simulink model "GitAffineFormationDelayInput"  (R2020b)
settings: Solver=ode4  StartTime=0.0  StopTime=50  FixedStep=0.01  RelTol=1e-3
(part 1 of 2)
settings Model: Creator=Fitz  LastModifiedBy=Fitz
settings DebuggingCC: UnderSpecifiedDimensionMsg=warning

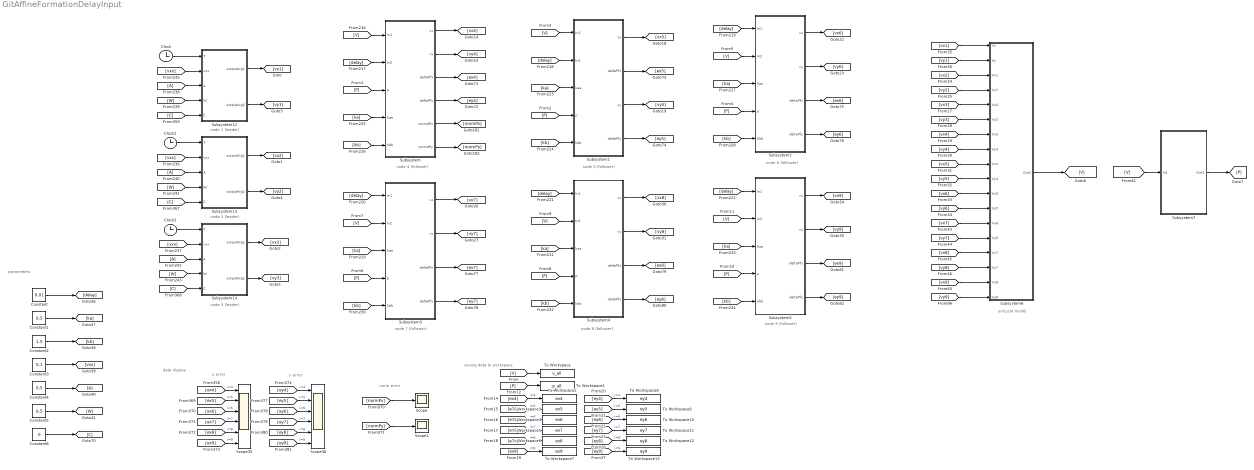
== system GitAffineFormationDelayInput ==
  note: unicycle model
  note: norm error
  note: y error
  note: x error
  note: node 1 (leader)
  note: data display
  note: parameters
  note: node 2 (leader)
  note: node 3 (leader)
  note: node 4 (follower)
  note: node 7 (follower)
  note: node 5 (follower)
  note: node 8 (follower)
  note: node 9 (follower)
  note: node 6 (follower)
  note: saving data to
      | workspace
  Clock : Clock
      settings: Decimation=100
  Clock1 : Clock
      settings: Decimation=100
  Clock2 : Clock
      settings: Decimation=100
  Constant : Constant  Value=0.01
  Constant1 : Constant  Value=0.5
  Constant2 : Constant  Value=1.5
  Constant3 : Constant  Value=0.1
  Constant4 : Constant  Value=0.5
  Constant5 : Constant  Value=0.5
  Constant6 : Constant  Value=0
  Scope : Scope
  Scope1 : Scope
  Scope35 : Scope  NumInputPorts=6
  Scope36 : Scope  NumInputPorts=6
  Subsystem : Subsystem
  Subsystem1 : Subsystem
  Subsystem12 : Subsystem
  Subsystem13 : Subsystem
  Subsystem14 : Subsystem
  Subsystem2 : Subsystem
  Subsystem3 : Subsystem
  Subsystem4 : Subsystem
  Subsystem5 : Subsystem
  Subsystem6 : Subsystem
  Subsystem7 : Subsystem
  To Workspace : ToWorkspace  VariableName=v_all  SaveFormat=Timeseries  SampleTime=-1
  To Workspace1 : ToWorkspace  VariableName=p_all  SaveFormat=Timeseries  SampleTime=-1
  To Workspace10 : ToWorkspace  VariableName=ey6  SaveFormat=Timeseries  SampleTime=-1
  To Workspace11 : ToWorkspace  VariableName=ey7  SaveFormat=Timeseries  SampleTime=-1
  To Workspace12 : ToWorkspace  VariableName=ey8  SaveFormat=Timeseries  SampleTime=-1
  To Workspace13 : ToWorkspace  VariableName=ey9  SaveFormat=Timeseries  SampleTime=-1
  To Workspace2 : ToWorkspace  VariableName=ex4  SaveFormat=Timeseries  SampleTime=-1
  To Workspace3 : ToWorkspace  VariableName=ex5  SaveFormat=Timeseries  SampleTime=-1
  To Workspace4 : ToWorkspace  VariableName=ex6  SaveFormat=Timeseries  SampleTime=-1
  To Workspace5 : ToWorkspace  VariableName=ex7  SaveFormat=Timeseries  SampleTime=-1
  To Workspace6 : ToWorkspace  VariableName=ex8  SaveFormat=Timeseries  SampleTime=-1
  To Workspace7 : ToWorkspace  VariableName=ex9  SaveFormat=Timeseries  SampleTime=-1
  To Workspace8 : ToWorkspace  VariableName=ey4  SaveFormat=Timeseries  SampleTime=-1
  To Workspace9 : ToWorkspace  VariableName=ey5  SaveFormat=Timeseries  SampleTime=-1
  wires:
  Constant/1 -> [delay]
  Constant1/1 -> [ka]
  Constant2/1 -> [kb]
  Constant3/1 -> [vxx]
  Constant4/1 -> [A]
  Constant5/1 -> [W]
  Constant6/1 -> [C]
  [ex4] -> Scope35/1  "i=4"
  [ex5] -> Scope35/2  "i=5"
  [ex6] -> Scope35/3  "i=6"
  [ex7] -> Scope35/4  "i=7"
  [ex8] -> Scope35/5  "i=8"
  [ex9] -> Scope35/6  "i=9"
  [ey9] -> Scope36/6  "i=9"
  [ey7] -> Scope36/4  "i=7"
  [ey5] -> Scope36/2  "i=5"
  [ey6] -> Scope36/3  "i=6"
  [ey8] -> Scope36/5  "i=8"
  [ey4] -> Scope36/1  "i=4"
  [V] -> Subsystem/1(In1)
  [delay] -> Subsystem/2(In2)
  [P] -> Subsystem/3(p)
  [ka] -> Subsystem/4(kaa)
  [kb] -> Subsystem/5(kbb)
  Subsystem/1(vx) -> [vx4]
  Subsystem/2(vy) -> [vy4]
  Subsystem/3(deltaPfx) -> [ex4]
  Subsystem/4(deltaPfy) -> [ey4]
  Subsystem/5(normdPx) -> [normPx]
  Subsystem/6(normdPy) -> [normPy]
  [V] -> Subsystem1/1(In1)
  [delay] -> Subsystem1/2(In2)
  [ka] -> Subsystem1/3(kaa)
  [P] -> Subsystem1/4(p)
  [kb] -> Subsystem1/5(kbb)
  Subsystem1/1(vx) -> [vx5]
  Subsystem1/2(deltaPfx) -> [ex5]
  Subsystem1/3(vy) -> [vy5]
  Subsystem1/4(deltaPfy) -> [ey5]
  [delay] -> Subsystem2/1(In1)
  [V] -> Subsystem2/2(In2)
  [ka] -> Subsystem2/3(kaa)
  [P] -> Subsystem2/4(p)
  [kb] -> Subsystem2/5(kbb)
  Subsystem2/1(vx) -> [vx6]
  Subsystem2/2(vy) -> [vy6]
  Subsystem2/3(deltaPfx) -> [ex6]
  Subsystem2/4(deltaPfy) -> [ey6]
  [delay] -> Subsystem3/1(In1)
  [V] -> Subsystem3/2(In2)
  [ka] -> Subsystem3/3(kaa)
  [P] -> Subsystem3/4(p)
  [kb] -> Subsystem3/5(kbb)
  Subsystem3/1(vx) -> [vx7]
  Subsystem3/2(vy) -> [vy7]
  Subsystem3/3(deltaPfx) -> [ex7]
  Subsystem3/4(deltaPfy) -> [ey7]
  [delay] -> Subsystem4/1(In1)
  [V] -> Subsystem4/2(In2)
  [ka] -> Subsystem4/3(kaa)
  [P] -> Subsystem4/4(p)
  [kb] -> Subsystem4/5(kbb)
  Subsystem4/1(vx) -> [vx8]
  Subsystem4/2(vy) -> [vy8]
  Subsystem4/3(deltaPfx) -> [ex8]
  Subsystem4/4(deltaPfy) -> [ey8]
  [delay] -> Subsystem5/1(In1)
  [V] -> Subsystem5/2(In2)
  [ka] -> Subsystem5/3(kaa)
  [P] -> Subsystem5/4(p)
  [kb] -> Subsystem5/5(kbb)
  Subsystem5/1(vx) -> [vx9]
  Subsystem5/2(vy) -> [vy9]
  Subsystem5/3(deltaPfx) -> [ex9]
  Subsystem5/4(deltaPfy) -> [ey9]
  Clock/1 -> Subsystem12/1(T)
  [vxx] -> Subsystem12/2(vxx)
  [A] -> Subsystem12/3(A)
  [W] -> Subsystem12/4(W)
  [C] -> Subsystem12/5(C)
  Subsystem12/1(outputArg1) -> [vx1]
  Subsystem12/2(outputArg2) -> [vy1]
  Clock1/1 -> Subsystem13/1(T)
  [vxx] -> Subsystem13/2(vxx)
  [A] -> Subsystem13/3(A)
  [W] -> Subsystem13/4(W)
  [C] -> Subsystem13/5(C)
  Subsystem13/1(outputArg1) -> [vx2]
  Subsystem13/2(outputArg2) -> [vy2]
  Clock2/1 -> Subsystem14/1(T)
  [vxx] -> Subsystem14/2(vxx)
  [A] -> Subsystem14/3(A)
  [W] -> Subsystem14/4(W)
  [C] -> Subsystem14/5(C)
  Subsystem14/1(outputArg1) -> [vx3]
  Subsystem14/2(outputArg2) -> [vy3]
  [normPx] -> Scope/1
  [normPy] -> Scope1/1
  [V] -> To Workspace/1
  [P] -> To Workspace1/1
  [ex4] -> To Workspace2/1  "i=4"
  [ex9] -> To Workspace7/1  "i=9"
  [ex8] -> To Workspace6/1  "i=8"
  [ex6] -> To Workspace4/1  "i=6"
  [ex5] -> To Workspace3/1  "i=5"
  [ex7] -> To Workspace5/1  "i=7"
  [ey4] -> To Workspace8/1  "i=4"
  [ey9] -> To Workspace13/1  "i=9"
  [ey8] -> To Workspace12/1  "i=8"
  [ey5] -> To Workspace9/1  "i=5"
  [ey6] -> To Workspace10/1  "i=6"
  [ey7] -> To Workspace11/1  "i=7"
  [vx1] -> Subsystem6/1(Vx)
  [vy1] -> Subsystem6/2(Vy)
  [vx2] -> Subsystem6/3(Vx1)
  [vy2] -> Subsystem6/4(Vy1)
  [vx3] -> Subsystem6/5(Vx2)
  [vy3] -> Subsystem6/6(Vy2)
  [vx4] -> Subsystem6/7(Vx3)
  [vy4] -> Subsystem6/8(Vy3)
  [vx5] -> Subsystem6/9(Vx4)
  [vy5] -> Subsystem6/10(Vy4)
  [vx6] -> Subsystem6/11(Vx5)
  [vy6] -> Subsystem6/12(Vy5)
  [vx7] -> Subsystem6/13(Vx6)
  [vy7] -> Subsystem6/14(Vy6)
  [vx8] -> Subsystem6/15(Vx7)
  [vy8] -> Subsystem6/16(Vy7)
  [vx9] -> Subsystem6/17(Vx8)
  [vy9] -> Subsystem6/18(Vy8)
  Subsystem6/1(Out1) -> [V]
  [V] -> Subsystem7/1(In1)
  Subsystem7/1(Out1) -> [P]

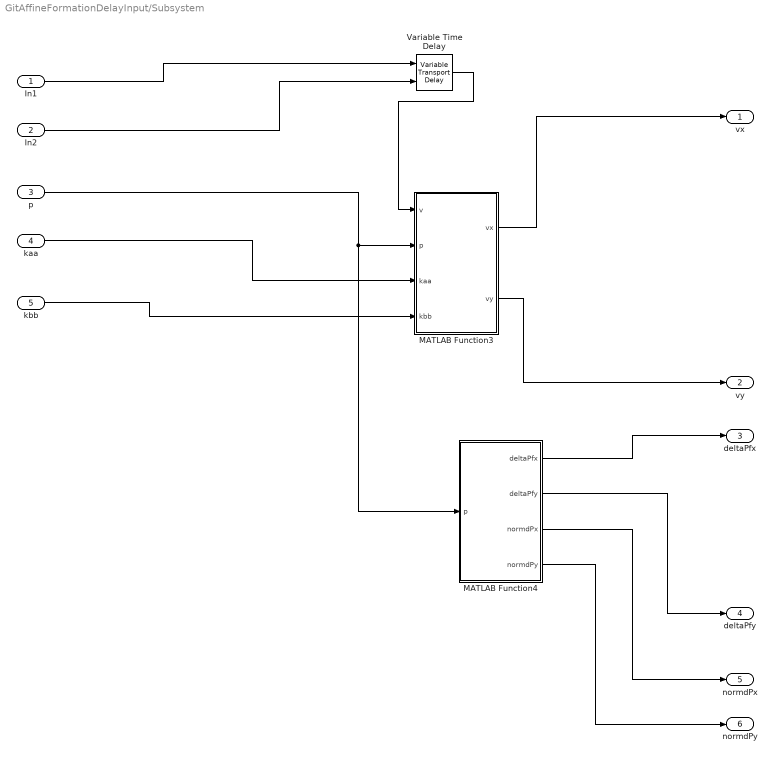
== system GitAffineFormationDelayInput/Subsystem ==
  In1 : Inport
  In2 : Inport  Port=2
  p : Inport  Port=3
  kaa : Inport  Port=4
  kbb : Inport  Port=5
  MATLAB Function3 : MATLAB Function  TreatAsAtomicUnit=on
  MATLAB Function4 : MATLAB Function  TreatAsAtomicUnit=on
  Variable Time Delay : VariableTransportDelay  MaximumDelay=10
  vx : Outport
  vy : Outport  Port=2
  deltaPfx : Outport  Port=3
  deltaPfy : Outport  Port=4
  normdPx : Outport  Port=5
  normdPy : Outport  Port=6
  wires:
  MATLAB Function4/2(deltaPfy) -> deltaPfy/1
  MATLAB Function4/1(deltaPfx) -> deltaPfx/1
  MATLAB Function3/2(vy) -> vy/1
  MATLAB Function3/1(vx) -> vx/1
  p/1 -> MATLAB Function4/1(p), MATLAB Function3/2(p)
  MATLAB Function4/3(normdPx) -> normdPx/1
  Variable Time Delay/1 -> MATLAB Function3/1(v)
  MATLAB Function4/4(normdPy) -> normdPy/1
  kbb/1 -> MATLAB Function3/4(kbb)
  In2/1 -> Variable Time Delay/2
  kaa/1 -> MATLAB Function3/3(kaa)
  In1/1 -> Variable Time Delay/1

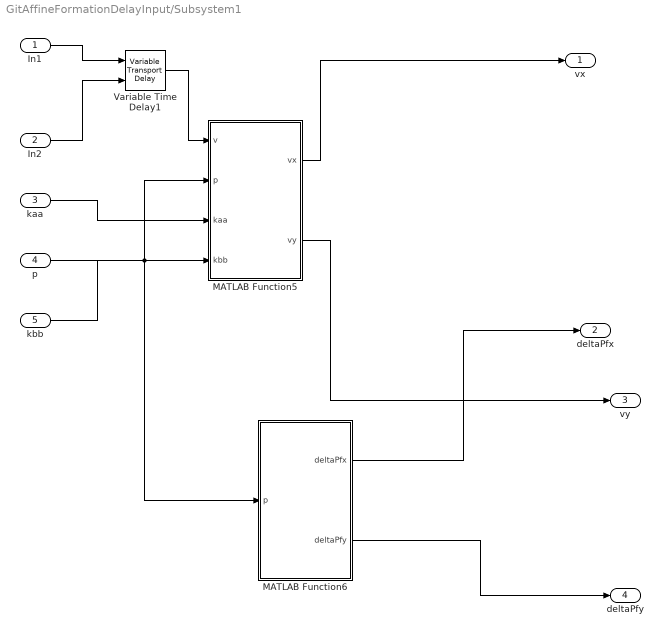
== system GitAffineFormationDelayInput/Subsystem1 ==
  In1 : Inport
  In2 : Inport  Port=2
  kaa : Inport  Port=3
  p : Inport  Port=4
  kbb : Inport  Port=5
  MATLAB Function5 : MATLAB Function  TreatAsAtomicUnit=on
  MATLAB Function6 : MATLAB Function  TreatAsAtomicUnit=on
  Variable Time Delay1 : VariableTransportDelay  MaximumDelay=10
  vx : Outport
  deltaPfx : Outport  Port=2
  vy : Outport  Port=3
  deltaPfy : Outport  Port=4
  wires:
  In1/1 -> Variable Time Delay1/1
  MATLAB Function5/2(vy) -> vy/1
  kbb/1 -> MATLAB Function5/4(kbb)
  p/1 -> MATLAB Function6/1(p), MATLAB Function5/2(p)
  kaa/1 -> MATLAB Function5/3(kaa)
  MATLAB Function5/1(vx) -> vx/1
  MATLAB Function6/1(deltaPfx) -> deltaPfx/1
  MATLAB Function6/2(deltaPfy) -> deltaPfy/1
  Variable Time Delay1/1 -> MATLAB Function5/1(v)
  In2/1 -> Variable Time Delay1/2

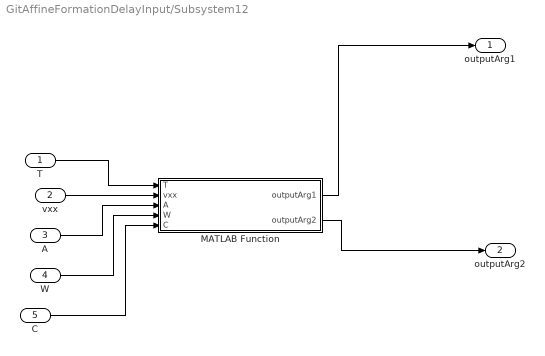
== system GitAffineFormationDelayInput/Subsystem12 ==
  T : Inport
  vxx : Inport  Port=2
  A : Inport  Port=3
  W : Inport  Port=4
  C : Inport  Port=5
  MATLAB Function : MATLAB Function  TreatAsAtomicUnit=on
  outputArg1 : Outport
  outputArg2 : Outport  Port=2
  wires:
  T/1 -> MATLAB Function/1(T)
  MATLAB Function/2(outputArg2) -> outputArg2/1
  C/1 -> MATLAB Function/5(C)
  MATLAB Function/1(outputArg1) -> outputArg1/1
  A/1 -> MATLAB Function/3(A)
  vxx/1 -> MATLAB Function/2(vxx)
  W/1 -> MATLAB Function/4(W)

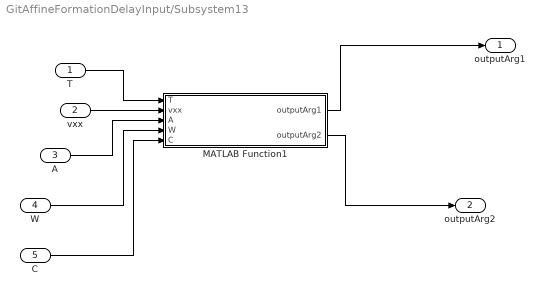
== system GitAffineFormationDelayInput/Subsystem13 ==
  T : Inport
  vxx : Inport  Port=2
  A : Inport  Port=3
  W : Inport  Port=4
  C : Inport  Port=5
  MATLAB Function1 : MATLAB Function  TreatAsAtomicUnit=on
  outputArg1 : Outport
  outputArg2 : Outport  Port=2
  wires:
  MATLAB Function1/1(outputArg1) -> outputArg1/1
  W/1 -> MATLAB Function1/4(W)
  vxx/1 -> MATLAB Function1/2(vxx)
  MATLAB Function1/2(outputArg2) -> outputArg2/1
  C/1 -> MATLAB Function1/5(C)
  T/1 -> MATLAB Function1/1(T)
  A/1 -> MATLAB Function1/3(A)

== system GitAffineFormationDelayInput/Subsystem14 ==
  T : Inport
  vxx : Inport  Port=2
  A : Inport  Port=3
  W : Inport  Port=4
  C : Inport  Port=5
  MATLAB Function2 : MATLAB Function  TreatAsAtomicUnit=on
  outputArg1 : Outport
  outputArg2 : Outport  Port=2
  wires:
  MATLAB Function2/1(outputArg1) -> outputArg1/1
  T/1 -> MATLAB Function2/1(T)
  MATLAB Function2/2(outputArg2) -> outputArg2/1
  vxx/1 -> MATLAB Function2/2(vxx)
  C/1 -> MATLAB Function2/5(C)
  A/1 -> MATLAB Function2/3(A)
  W/1 -> MATLAB Function2/4(W)

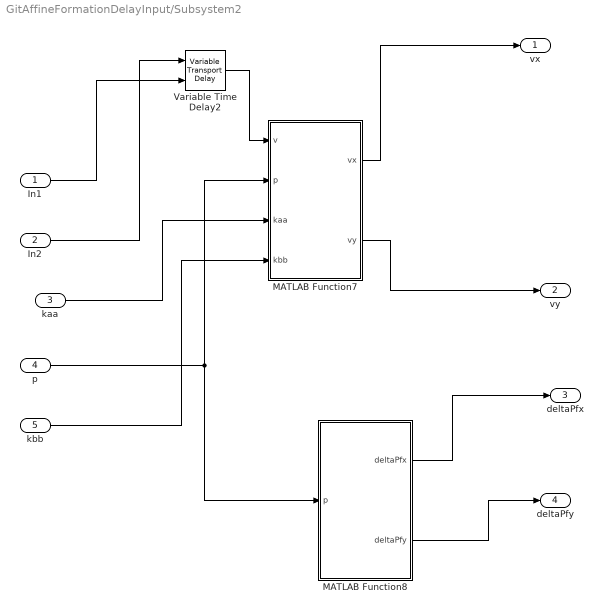
== system GitAffineFormationDelayInput/Subsystem2 ==
  In1 : Inport
  In2 : Inport  Port=2
  kaa : Inport  Port=3
  p : Inport  Port=4
  kbb : Inport  Port=5
  MATLAB Function7 : MATLAB Function  TreatAsAtomicUnit=on
  MATLAB Function8 : MATLAB Function  TreatAsAtomicUnit=on
  Variable Time Delay2 : VariableTransportDelay  MaximumDelay=10
  vx : Outport
  vy : Outport  Port=2
  deltaPfx : Outport  Port=3
  deltaPfy : Outport  Port=4
  wires:
  kbb/1 -> MATLAB Function7/4(kbb)
  MATLAB Function7/1(vx) -> vx/1
  Variable Time Delay2/1 -> MATLAB Function7/1(v)
  MATLAB Function7/2(vy) -> vy/1
  p/1 -> MATLAB Function8/1(p), MATLAB Function7/2(p)
  MATLAB Function8/1(deltaPfx) -> deltaPfx/1
  kaa/1 -> MATLAB Function7/3(kaa)
  MATLAB Function8/2(deltaPfy) -> deltaPfy/1
  In2/1 -> Variable Time Delay2/1
  In1/1 -> Variable Time Delay2/2

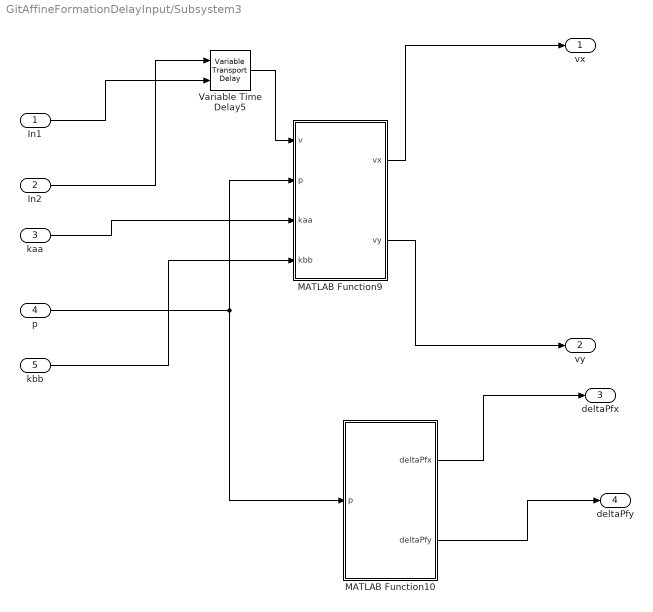
== system GitAffineFormationDelayInput/Subsystem3 ==
  In1 : Inport
  In2 : Inport  Port=2
  kaa : Inport  Port=3
  p : Inport  Port=4
  kbb : Inport  Port=5
  MATLAB Function10 : MATLAB Function  TreatAsAtomicUnit=on
  MATLAB Function9 : MATLAB Function  TreatAsAtomicUnit=on
  Variable Time Delay5 : VariableTransportDelay  MaximumDelay=10
  vx : Outport
  vy : Outport  Port=2
  deltaPfx : Outport  Port=3
  deltaPfy : Outport  Port=4
  wires:
  MATLAB Function9/2(vy) -> vy/1
  p/1 -> MATLAB Function10/1(p), MATLAB Function9/2(p)
  kbb/1 -> MATLAB Function9/4(kbb)
  MATLAB Function9/1(vx) -> vx/1
  In2/1 -> Variable Time Delay5/1
  kaa/1 -> MATLAB Function9/3(kaa)
  Variable Time Delay5/1 -> MATLAB Function9/1(v)
  In1/1 -> Variable Time Delay5/2
  MATLAB Function10/1(deltaPfx) -> deltaPfx/1
  MATLAB Function10/2(deltaPfy) -> deltaPfy/1

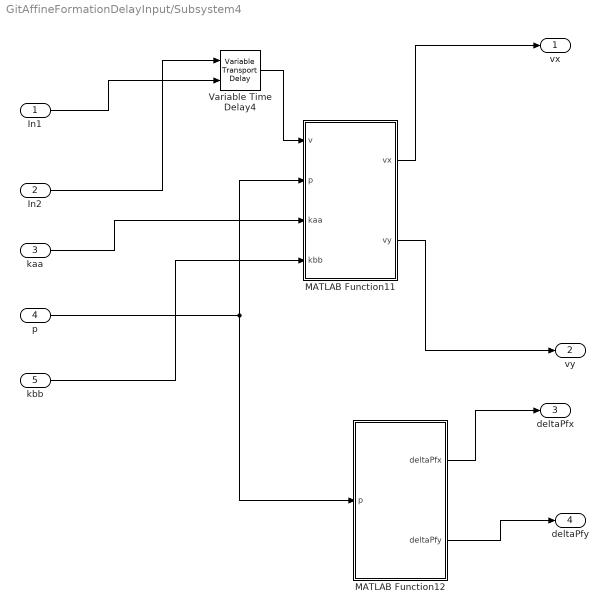
== system GitAffineFormationDelayInput/Subsystem4 ==
  In1 : Inport
  In2 : Inport  Port=2
  kaa : Inport  Port=3
  p : Inport  Port=4
  kbb : Inport  Port=5
  MATLAB Function11 : MATLAB Function  TreatAsAtomicUnit=on
  MATLAB Function12 : MATLAB Function  TreatAsAtomicUnit=on
  Variable Time Delay4 : VariableTransportDelay  MaximumDelay=10
  vx : Outport
  vy : Outport  Port=2
  deltaPfx : Outport  Port=3
  deltaPfy : Outport  Port=4
  wires:
  MATLAB Function12/1(deltaPfx) -> deltaPfx/1
  MATLAB Function11/1(vx) -> vx/1
  Variable Time Delay4/1 -> MATLAB Function11/1(v)
  MATLAB Function11/2(vy) -> vy/1
  p/1 -> MATLAB Function12/1(p), MATLAB Function11/2(p)
  MATLAB Function12/2(deltaPfy) -> deltaPfy/1
  In1/1 -> Variable Time Delay4/2
  kbb/1 -> MATLAB Function11/4(kbb)
  kaa/1 -> MATLAB Function11/3(kaa)
  In2/1 -> Variable Time Delay4/1

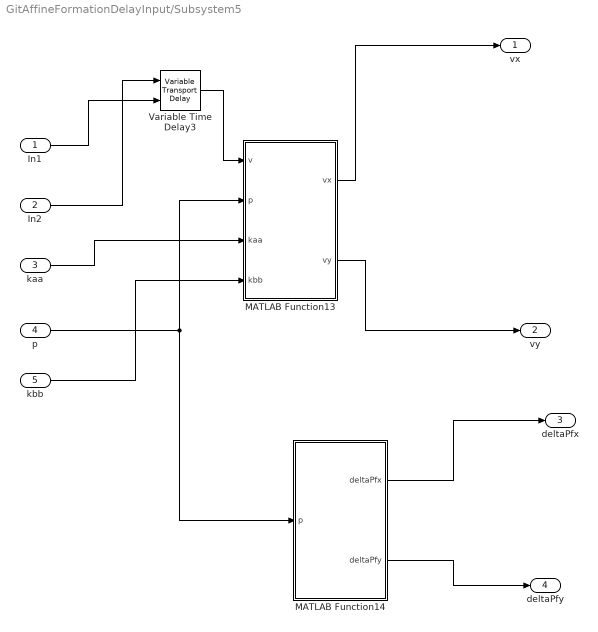
== system GitAffineFormationDelayInput/Subsystem5 ==
  In1 : Inport
  In2 : Inport  Port=2
  kaa : Inport  Port=3
  p : Inport  Port=4
  kbb : Inport  Port=5
  MATLAB Function13 : MATLAB Function  TreatAsAtomicUnit=on
  MATLAB Function14 : MATLAB Function  TreatAsAtomicUnit=on
  Variable Time Delay3 : VariableTransportDelay  MaximumDelay=10
  vx : Outport
  vy : Outport  Port=2
  deltaPfx : Outport  Port=3
  deltaPfy : Outport  Port=4
  wires:
  p/1 -> MATLAB Function14/1(p), MATLAB Function13/2(p)
  MATLAB Function13/1(vx) -> vx/1
  MATLAB Function13/2(vy) -> vy/1
  Variable Time Delay3/1 -> MATLAB Function13/1(v)
  kbb/1 -> MATLAB Function13/4(kbb)
  kaa/1 -> MATLAB Function13/3(kaa)
  MATLAB Function14/2(deltaPfy) -> deltaPfy/1
  In1/1 -> Variable Time Delay3/2
  MATLAB Function14/1(deltaPfx) -> deltaPfx/1
  In2/1 -> Variable Time Delay3/1

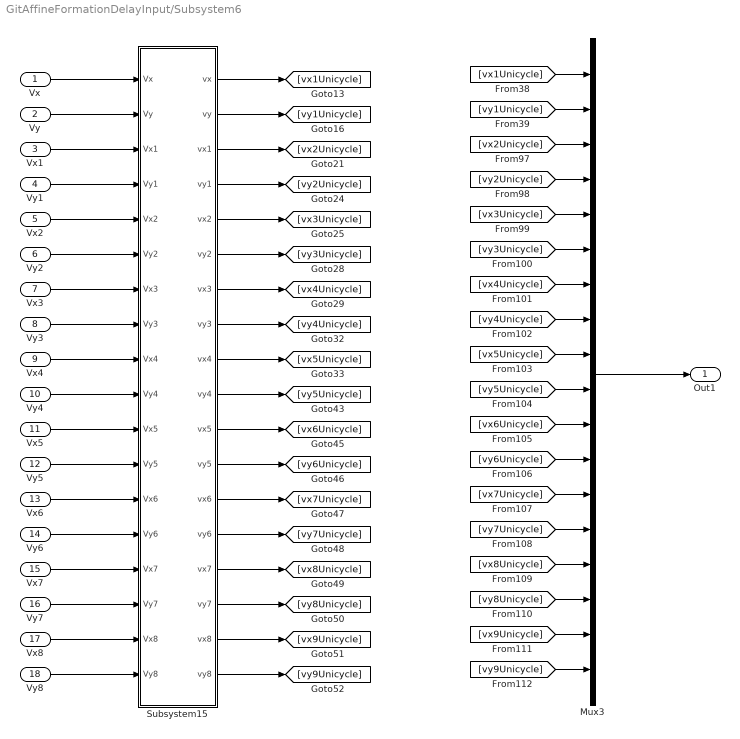
== system GitAffineFormationDelayInput/Subsystem6 ==
  Vx : Inport
  Vy : Inport  Port=2
  Vx1 : Inport  Port=3
  Vy1 : Inport  Port=4
  Vx2 : Inport  Port=5
  Vy2 : Inport  Port=6
  Vx3 : Inport  Port=7
  Vy3 : Inport  Port=8
  Vx4 : Inport  Port=9
  Vy4 : Inport  Port=10
  Vx5 : Inport  Port=11
  Vy5 : Inport  Port=12
  Vx6 : Inport  Port=13
  Vy6 : Inport  Port=14
  Vx7 : Inport  Port=15
  Vy7 : Inport  Port=16
  Vx8 : Inport  Port=17
  Vy8 : Inport  Port=18
  Mux3 : Mux  Inputs=18
  Subsystem15 : Subsystem
  Out1 : Outport
  wires:
  Vx8/1 -> Subsystem15/17(Vx8)
  Subsystem15/18(vy8) -> [vy9Unicycle]
  Subsystem15/5(vx2) -> [vx3Unicycle]
  Vx4/1 -> Subsystem15/9(Vx4)
  Subsystem15/1(vx) -> [vx1Unicycle]
  [vy5Unicycle] -> Mux3/10
  Subsystem15/17(vx8) -> [vx9Unicycle]
  Vy7/1 -> Subsystem15/16(Vy7)
  [vx5Unicycle] -> Mux3/9
  Subsystem15/15(vx7) -> [vx8Unicycle]
  Subsystem15/9(vx4) -> [vx5Unicycle]
  Subsystem15/14(vy6) -> [vy7Unicycle]
  Subsystem15/13(vx6) -> [vx7Unicycle]
  Vy8/1 -> Subsystem15/18(Vy8)
  Subsystem15/12(vy5) -> [vy6Unicycle]
  Subsystem15/2(vy) -> [vy1Unicycle]
  Subsystem15/4(vy1) -> [vy2Unicycle]
  Vx2/1 -> Subsystem15/5(Vx2)
  Subsystem15/16(vy7) -> [vy8Unicycle]
  Vy6/1 -> Subsystem15/14(Vy6)
  Vx6/1 -> Subsystem15/13(Vx6)
  [vy4Unicycle] -> Mux3/8
  [vy1Unicycle] -> Mux3/2
  Subsystem15/7(vx3) -> [vx4Unicycle]
  [vy3Unicycle] -> Mux3/6
  [vx9Unicycle] -> Mux3/17
  [vx8Unicycle] -> Mux3/15
  [vx7Unicycle] -> Mux3/13
  Vy1/1 -> Subsystem15/4(Vy1)
  Vx7/1 -> Subsystem15/15(Vx7)
  [vx3Unicycle] -> Mux3/5
  [vy6Unicycle] -> Mux3/12
  Subsystem15/6(vy2) -> [vy3Unicycle]
  Vy3/1 -> Subsystem15/8(Vy3)
  Subsystem15/8(vy3) -> [vy4Unicycle]
  Vy4/1 -> Subsystem15/10(Vy4)
  [vx6Unicycle] -> Mux3/11
  Subsystem15/3(vx1) -> [vx2Unicycle]
  Vy2/1 -> Subsystem15/6(Vy2)
  [vx1Unicycle] -> Mux3/1
  [vy7Unicycle] -> Mux3/14
  Subsystem15/10(vy4) -> [vy5Unicycle]
  Subsystem15/11(vx5) -> [vx6Unicycle]
  [vx4Unicycle] -> Mux3/7
  Vx/1 -> Subsystem15/1(Vx)
  [vx2Unicycle] -> Mux3/3
  [vy2Unicycle] -> Mux3/4
  [vy8Unicycle] -> Mux3/16
  [vy9Unicycle] -> Mux3/18
  Vx3/1 -> Subsystem15/7(Vx3)
  Vx1/1 -> Subsystem15/3(Vx1)
  Vx5/1 -> Subsystem15/11(Vx5)
  Vy/1 -> Subsystem15/2(Vy)
  Vy5/1 -> Subsystem15/12(Vy5)
  Mux3/1 -> Out1/1

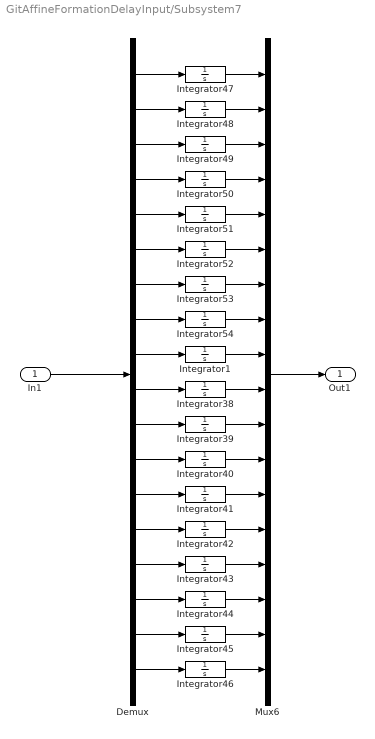
== system GitAffineFormationDelayInput/Subsystem7 ==
  In1 : Inport
  Demux : Demux  Outputs=18
  Integrator1 : Integrator  InitialCondition=-1
  Integrator38 : Integrator  InitialCondition=-2.2
  Integrator{39,43,49..51,53} (6 alike) : Integrator  InitialCondition=1
  Integrator40 : Integrator  InitialCondition=3
  Integrator41 : Integrator  InitialCondition=-3
  Integrator42 : Integrator  InitialCondition=-3
  Integrator44 : Integrator  InitialCondition=3.5
  Integrator45 : Integrator  InitialCondition=-5
  Integrator46 : Integrator  InitialCondition=-3.5
  Integrator47 : Integrator  InitialCondition=2
  Integrator48 : Integrator
  Integrator52 : Integrator  InitialCondition=-1
  Integrator54 : Integrator  InitialCondition=2.2
  Mux6 : Mux  Inputs=18
  Out1 : Outport
  wires:
  Demux/3 -> Integrator49/1
  Demux/6 -> Integrator52/1
  Demux/2 -> Integrator48/1
  Mux6/1 -> Out1/1
  Demux/9 -> Integrator1/1
  Integrator49/1 -> Mux6/3
  Integrator43/1 -> Mux6/15
  Demux/14 -> Integrator42/1
  Demux/16 -> Integrator44/1
  Demux/12 -> Integrator40/1
  Demux/4 -> Integrator50/1
  Integrator54/1 -> Mux6/8
  Demux/10 -> Integrator38/1
  Integrator47/1 -> Mux6/1
  Integrator1/1 -> Mux6/9
  Demux/17 -> Integrator45/1
  Integrator45/1 -> Mux6/17
  Demux/18 -> Integrator46/1
  Demux/5 -> Integrator51/1
  Demux/13 -> Integrator41/1
  Integrator38/1 -> Mux6/10
  Integrator48/1 -> Mux6/2
  Integrator41/1 -> Mux6/13
  Integrator39/1 -> Mux6/11
  Integrator46/1 -> Mux6/18
  Demux/11 -> Integrator39/1
  In1/1 -> Demux/1
  Demux/8 -> Integrator54/1
  Integrator44/1 -> Mux6/16
  Integrator52/1 -> Mux6/6
  Integrator51/1 -> Mux6/5
  Integrator40/1 -> Mux6/12
  Demux/1 -> Integrator47/1
  Integrator53/1 -> Mux6/7
  Demux/7 -> Integrator53/1
  Integrator42/1 -> Mux6/14
  Integrator50/1 -> Mux6/4
  Demux/15 -> Integrator43/1

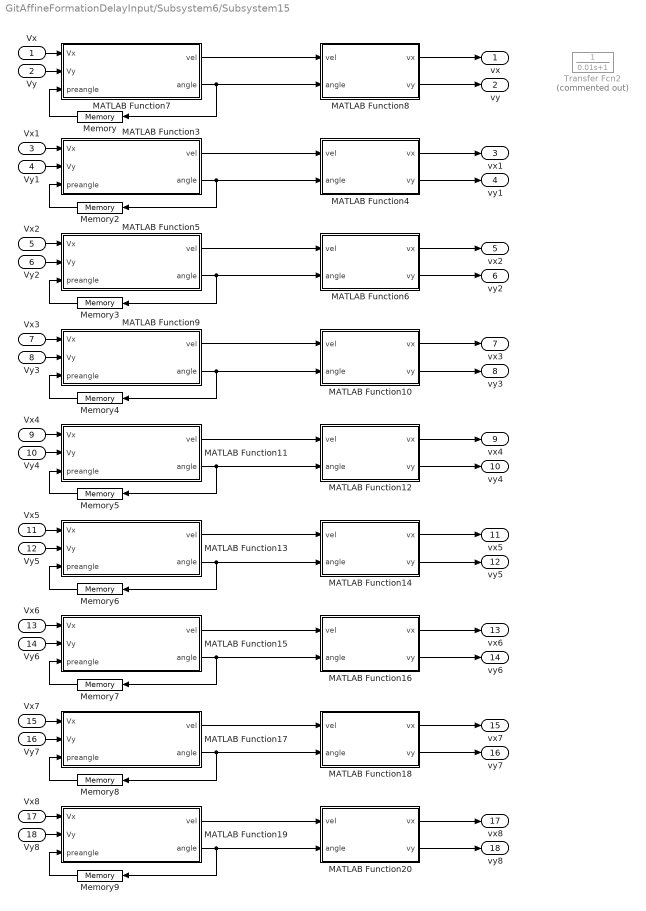
== system GitAffineFormationDelayInput/Subsystem6/Subsystem15 ==
  Vx : Inport
  Vy : Inport  Port=2
  Vx1 : Inport  Port=3
  Vy1 : Inport  Port=4
  Vx2 : Inport  Port=5
  Vy2 : Inport  Port=6
  Vx3 : Inport  Port=7
  Vy3 : Inport  Port=8
  Vx4 : Inport  Port=9
  Vy4 : Inport  Port=10
  Vx5 : Inport  Port=11
  Vy5 : Inport  Port=12
  Vx6 : Inport  Port=13
  Vy6 : Inport  Port=14
  Vx7 : Inport  Port=15
  Vy7 : Inport  Port=16
  Vx8 : Inport  Port=17
  Vy8 : Inport  Port=18
  MATLAB Function10 : MATLAB Function  TreatAsAtomicUnit=on
  MATLAB Function11 : MATLAB Function  TreatAsAtomicUnit=on
  MATLAB Function12 : MATLAB Function  TreatAsAtomicUnit=on
  MATLAB Function13 : MATLAB Function  TreatAsAtomicUnit=on
  MATLAB Function14 : MATLAB Function  TreatAsAtomicUnit=on
  MATLAB Function15 : MATLAB Function  TreatAsAtomicUnit=on
  MATLAB Function16 : MATLAB Function  TreatAsAtomicUnit=on
  MATLAB Function17 : MATLAB Function  TreatAsAtomicUnit=on
  MATLAB Function18 : MATLAB Function  TreatAsAtomicUnit=on
  MATLAB Function19 : MATLAB Function  TreatAsAtomicUnit=on
  MATLAB Function20 : MATLAB Function  TreatAsAtomicUnit=on
  MATLAB Function3 : MATLAB Function  TreatAsAtomicUnit=on
  MATLAB Function4 : MATLAB Function  TreatAsAtomicUnit=on
  MATLAB Function5 : MATLAB Function  TreatAsAtomicUnit=on
  MATLAB Function6 : MATLAB Function  TreatAsAtomicUnit=on
  MATLAB Function7 : MATLAB Function  TreatAsAtomicUnit=on
  MATLAB Function8 : MATLAB Function  TreatAsAtomicUnit=on
  MATLAB Function9 : MATLAB Function  TreatAsAtomicUnit=on
  Memory{,2..9} (9 alike) : Memory
  Transfer Fcn2 : TransferFcn  Commented=on  Denominator=[0.01 1]
  vx : Outport
  vy : Outport  Port=2
  vx1 : Outport  Port=3
  vy1 : Outport  Port=4
  vx2 : Outport  Port=5
  vy2 : Outport  Port=6
  vx3 : Outport  Port=7
  vy3 : Outport  Port=8
  vx4 : Outport  Port=9
  vy4 : Outport  Port=10
  vx5 : Outport  Port=11
  vy5 : Outport  Port=12
  vx6 : Outport  Port=13
  vy6 : Outport  Port=14
  vx7 : Outport  Port=15
  vy7 : Outport  Port=16
  vx8 : Outport  Port=17
  vy8 : Outport  Port=18
  wires:
  MATLAB Function8/2(vy) -> vy/1
  MATLAB Function6/2(vy) -> vy2/1
  MATLAB Function9/1(vel) -> MATLAB Function10/1(vel)
  MATLAB Function4/2(vy) -> vy1/1
  MATLAB Function19/2(angle) -> MATLAB Function20/2(angle), Memory9/1
  Vy3/1 -> MATLAB Function9/2(Vy)
  Memory7/1 -> MATLAB Function15/3(preangle)
  MATLAB Function15/2(angle) -> MATLAB Function16/2(angle), Memory7/1
  MATLAB Function10/1(vx) -> vx3/1
  Memory4/1 -> MATLAB Function9/3(preangle)
  MATLAB Function9/2(angle) -> MATLAB Function10/2(angle), Memory4/1
  Memory3/1 -> MATLAB Function5/3(preangle)
  Memory9/1 -> MATLAB Function19/3(preangle)
  Memory2/1 -> MATLAB Function3/3(preangle)
  Memory6/1 -> MATLAB Function13/3(preangle)
  MATLAB Function3/2(angle) -> MATLAB Function4/2(angle), Memory2/1
  MATLAB Function11/1(vel) -> MATLAB Function12/1(vel)
  MATLAB Function3/1(vel) -> MATLAB Function4/1(vel)
  Vy/1 -> MATLAB Function7/2(Vy)
  MATLAB Function20/2(vy) -> vy8/1
  MATLAB Function15/1(vel) -> MATLAB Function16/1(vel)
  Vx/1 -> MATLAB Function7/1(Vx)
  Memory/1 -> MATLAB Function7/3(preangle)
  Memory8/1 -> MATLAB Function17/3(preangle)
  MATLAB Function19/1(vel) -> MATLAB Function20/1(vel)
  MATLAB Function17/2(angle) -> MATLAB Function18/2(angle), Memory8/1
  MATLAB Function5/2(angle) -> MATLAB Function6/2(angle), Memory3/1
  MATLAB Function5/1(vel) -> MATLAB Function6/1(vel)
  Vx8/1 -> MATLAB Function19/1(Vx)
  Vy8/1 -> MATLAB Function19/2(Vy)
  MATLAB Function13/2(angle) -> MATLAB Function14/2(angle), Memory6/1
  MATLAB Function17/1(vel) -> MATLAB Function18/1(vel)
  MATLAB Function18/1(vx) -> vx7/1
  Memory5/1 -> MATLAB Function11/3(preangle)
  Vx2/1 -> MATLAB Function5/1(Vx)
  MATLAB Function13/1(vel) -> MATLAB Function14/1(vel)
  MATLAB Function8/1(vx) -> vx/1
  Vy1/1 -> MATLAB Function3/2(Vy)
  MATLAB Function11/2(angle) -> MATLAB Function12/2(angle), Memory5/1
  Vx1/1 -> MATLAB Function3/1(Vx)
  MATLAB Function6/1(vx) -> vx2/1
  Vy4/1 -> MATLAB Function11/2(Vy)
  MATLAB Function18/2(vy) -> vy7/1
  Vx3/1 -> MATLAB Function9/1(Vx)
  Vx7/1 -> MATLAB Function17/1(Vx)
  MATLAB Function12/2(vy) -> vy4/1
  Vy7/1 -> MATLAB Function17/2(Vy)
  MATLAB Function10/2(vy) -> vy3/1
  MATLAB Function12/1(vx) -> vx4/1
  MATLAB Function4/1(vx) -> vx1/1
  Vy6/1 -> MATLAB Function15/2(Vy)
  MATLAB Function20/1(vx) -> vx8/1
  Vx4/1 -> MATLAB Function11/1(Vx)
  MATLAB Function16/1(vx) -> vx6/1
  Vx6/1 -> MATLAB Function15/1(Vx)
  MATLAB Function16/2(vy) -> vy6/1
  Vy2/1 -> MATLAB Function5/2(Vy)
  Vy5/1 -> MATLAB Function13/2(Vy)
  Vx5/1 -> MATLAB Function13/1(Vx)
  MATLAB Function14/1(vx) -> vx5/1
  MATLAB Function14/2(vy) -> vy5/1
  MATLAB Function7/1(vel) -> MATLAB Function8/1(vel)
  MATLAB Function7/2(angle) -> MATLAB Function8/2(angle), Memory/1

== matlab function GitAffineFormationDelayInput/Subsystem/MATLAB Function4 ==
  data: deltaPfx output; p input; deltaPfy output; normdPx output; normdPy output
function [deltaPfx,deltaPfy,normdPx,normdPy]  = fcn_errorV4(p)

leaderNum=3;
dim=2;
stressMat=[-0.438878870659884,0.292585913773256,0.292585913773256,0,0,0,0,-0.0731464784433140,-0.0731464784433141;0.292585913773256,-0.615360326958201,0,0.420303051109364,-0.0673401385127307,0,-0.0301884994116881,0,0;0.292585913773256,0,-0.615360326958201,-0.0673401385127306,0.420303051109363,-0.0301884994116881,0,0,0;0,0.420303051109364,-0.0673401385127306,-0.703215455187769,-0.00271037000549659,0.352962912596633,0,0,0;0,-0.0673401385127307,0.420303051109363,-0.00271037000549659,-0.703215455187768,0,0.352962912596632,0,0;0,0,-0.0301884994116881,0.352962912596633,0,-0.607698639186239,-0.00766168777196264,0.292585913773257,0;0,-0.0301884994116881,0,0,0.352962912596632,-0.00766168777196264,-0.607698639186238,0,0.292585913773256;-0.0731464784433140,0,0,0,0,0.292585913773257,0,-0.402305631438228,0.182866196108285;-0.0731464784433141,0,0,0,0,0,0.292585913773256,0.182866196108285,-0.402305631438227];

stressMat_ff=stressMat(leaderNum+1:end,leaderNum+1:end);
stressMat_fl=stressMat(leaderNum+1:end,1:leaderNum);

p_all = p;
p_ell=p_all(1:dim*leaderNum);
p_f=p_all(dim*leaderNum+1:end);


delta=p_f+(kron(stressMat_ff,eye(dim)))\kron(stressMat_fl,eye(dim))*p_ell;
%deltaPf=delta(1,1)+delta(2,1);
deltaPfx=delta(1,1);
deltaPfy=delta(2,1);
ax=[delta(1,1),delta(3,1),delta(5,1),delta(7,1),delta(9,1),delta(11,1)];
ay=[delta(2,1),delta(4,1),delta(6,1),delta(8,1),delta(10,1),delta(12,1)];
normdPx=norm(ax);
normdPy=norm(ay);

== matlab function GitAffineFormationDelayInput/Subsystem3/MATLAB Function9 ==
  data: v input; vx output size=1; p input; vy output size=1; kaa input; kbb input
function [vx,vy] = fcn_followerV4(v,p,kaa,kbb)

reV=zeros(2,9);
reP=zeros(2,9);
reV=reshape(v,2,9);
reP=reshape(p,2,9);

ka=kaa;
kb=kbb;
vx7=0;
vy7=0;
nodenum=9;
leaderNum=3;
neighborMat=zeros(nodenum,nodenum);
neighborMat(1,2)=1;neighborMat(1,3)=1;neighborMat(1,8)=1;neighborMat(1,9)=1;
neighborMat(2,4)=1;neighborMat(2,7)=1;
neighborMat(3,5)=1;neighborMat(3,6)=1;neighborMat(3,4)=1;neighborMat(2,5)=1;
neighborMat(4,5)=1;neighborMat(4,6)=1;neighborMat(2,7)=1;neighborMat(4,7)=0;
neighborMat(5,7)=1;neighborMat(5,8)=0;neighborMat(5,6)=0;
neighborMat(6,7)=1;neighborMat(6,8)=1;
neighborMat(7,9)=1;
neighborMat(8,9)=1;
m=sum(sum(neighborMat)); % number of edges
neighborMat=neighborMat+neighborMat';
stressMat=[-0.438878870659884,0.292585913773256,0.292585913773256,0,0,0,0,-0.0731464784433140,-0.0731464784433141;0.292585913773256,-0.615360326958201,0,0.420303051109364,-0.0673401385127307,0,-0.0301884994116881,0,0;0.292585913773256,0,-0.615360326958201,-0.0673401385127306,0.420303051109363,-0.0301884994116881,0,0,0;0,0.420303051109364,-0.0673401385127306,-0.703215455187769,-0.00271037000549659,0.352962912596633,0,0,0;0,-0.0673401385127307,0.420303051109363,-0.00271037000549659,-0.703215455187768,0,0.352962912596632,0,0;0,0,-0.0301884994116881,0.352962912596633,0,-0.607698639186239,-0.00766168777196264,0.292585913773257,0;0,-0.0301884994116881,0,0,0.352962912596632,-0.00766168777196264,-0.607698639186238,0,0.292585913773256;-0.0731464784433140,0,0,0,0,0.292585913773257,0,-0.402305631438228,0.182866196108285;-0.0731464784433141,0,0,0,0,0,0.292585913773256,0.182866196108285,-0.402305631438227];

stressMat_ff=stressMat(leaderNum+1:end,leaderNum+1:end);

for j=1:nodenum 
    if neighborMat(7,j)==1 && j~=7
        omegaij=stressMat(7,j);
        vx7=vx7-ka*kb*omegaij*(reP(1,7)-reP(1,j))-kb*omegaij*(reV(1,7)-reV(1,j));
        vy7=vy7-ka*kb*omegaij*(reP(2,7)-reP(2,j))-kb*omegaij*(reV(2,7)-reV(2,j));
    end
end
vx7=vx7+reV(1,7);
vy7=vy7+reV(2,7);

vx = vx7;
vy = vy7;

== matlab function GitAffineFormationDelayInput/Subsystem4/MATLAB Function11 ==
  data: v input; vx output size=1; p input; vy output size=1; kaa input; kbb input
function [vx,vy] = fcn_followerV4(v,p,kaa,kbb)

reV=zeros(2,9);
reP=zeros(2,9);
reV=reshape(v,2,9);
reP=reshape(p,2,9);
ka=kaa;
%kb=1.0425;
kb=kbb;
vx8=0;
vy8=0;
nodenum=9;
leaderNum=3;
neighborMat=zeros(nodenum,nodenum);
neighborMat(1,2)=1;neighborMat(1,3)=1;neighborMat(1,8)=1;neighborMat(1,9)=1;
neighborMat(2,4)=1;neighborMat(2,7)=1;
neighborMat(3,5)=1;neighborMat(3,6)=1;neighborMat(3,4)=1;neighborMat(2,5)=1;
neighborMat(4,5)=1;neighborMat(4,6)=1;neighborMat(2,7)=1;neighborMat(4,7)=0;
neighborMat(5,7)=1;neighborMat(5,8)=0;neighborMat(5,6)=0;
neighborMat(6,7)=1;neighborMat(6,8)=1;
neighborMat(7,9)=1;
neighborMat(8,9)=1;
m=sum(sum(neighborMat)); % number of edges
neighborMat=neighborMat+neighborMat';
stressMat=[-0.438878870659884,0.292585913773256,0.292585913773256,0,0,0,0,-0.0731464784433140,-0.0731464784433141;0.292585913773256,-0.615360326958201,0,0.420303051109364,-0.0673401385127307,0,-0.0301884994116881,0,0;0.292585913773256,0,-0.615360326958201,-0.0673401385127306,0.420303051109363,-0.0301884994116881,0,0,0;0,0.420303051109364,-0.0673401385127306,-0.703215455187769,-0.00271037000549659,0.352962912596633,0,0,0;0,-0.0673401385127307,0.420303051109363,-0.00271037000549659,-0.703215455187768,0,0.352962912596632,0,0;0,0,-0.0301884994116881,0.352962912596633,0,-0.607698639186239,-0.00766168777196264,0.292585913773257,0;0,-0.0301884994116881,0,0,0.352962912596632,-0.00766168777196264,-0.607698639186238,0,0.292585913773256;-0.0731464784433140,0,0,0,0,0.292585913773257,0,-0.402305631438228,0.182866196108285;-0.0731464784433141,0,0,0,0,0,0.292585913773256,0.182866196108285,-0.402305631438227];


for j=1:nodenum 
    if neighborMat(8,j)==1 && j~=8
        omegaij=stressMat(8,j);
        vx8=vx8-ka*kb*omegaij*(reP(1,8)-reP(1,j))-kb*omegaij*(reV(1,8)-reV(1,j));
        vy8=vy8-ka*kb*omegaij*(reP(2,8)-reP(2,j))-kb*omegaij*(reV(2,8)-reV(2,j));
    end
end
vx8=vx8+reV(1,8);
vy8=vy8+reV(2,8);

vx = vx8;
vy = vy8;

== matlab function GitAffineFormationDelayInput/Subsystem1/MATLAB Function5 ==
  data: v input; vx output size=1; p input; vy output size=1; kaa input; kbb input
function [vx,vy] = fcn_followerV4(v,p,kaa,kbb)

reV=zeros(2,9);
reP=zeros(2,9);
reV=reshape(v,2,9);
reP=reshape(p,2,9);

ka=kaa;
kb=kbb;
vx5=0;
vy5=0;

nodenum=9;
leaderNum=3;
neighborMat=zeros(nodenum,nodenum);
neighborMat(1,2)=1;neighborMat(1,3)=1;neighborMat(1,8)=1;neighborMat(1,9)=1;
neighborMat(2,4)=1;neighborMat(2,7)=1;
neighborMat(3,5)=1;neighborMat(3,6)=1;neighborMat(3,4)=1;neighborMat(2,5)=1;
neighborMat(4,5)=1;neighborMat(4,6)=1;neighborMat(2,7)=1;neighborMat(4,7)=0;
neighborMat(5,7)=1;neighborMat(5,8)=0;neighborMat(5,6)=0;
neighborMat(6,7)=1;neighborMat(6,8)=1;
neighborMat(7,9)=1;
neighborMat(8,9)=1;
m=sum(sum(neighborMat)); % number of edges
neighborMat=neighborMat+neighborMat';
stressMat=[-0.438878870659884,0.292585913773256,0.292585913773256,0,0,0,0,-0.0731464784433140,-0.0731464784433141;0.292585913773256,-0.615360326958201,0,0.420303051109364,-0.0673401385127307,0,-0.0301884994116881,0,0;0.292585913773256,0,-0.615360326958201,-0.0673401385127306,0.420303051109363,-0.0301884994116881,0,0,0;0,0.420303051109364,-0.0673401385127306,-0.703215455187769,-0.00271037000549659,0.352962912596633,0,0,0;0,-0.0673401385127307,0.420303051109363,-0.00271037000549659,-0.703215455187768,0,0.352962912596632,0,0;0,0,-0.0301884994116881,0.352962912596633,0,-0.607698639186239,-0.00766168777196264,0.292585913773257,0;0,-0.0301884994116881,0,0,0.352962912596632,-0.00766168777196264,-0.607698639186238,0,0.292585913773256;-0.0731464784433140,0,0,0,0,0.292585913773257,0,-0.402305631438228,0.182866196108285;-0.0731464784433141,0,0,0,0,0,0.292585913773256,0.182866196108285,-0.402305631438227];

%%
for j=1:nodenum 
    if neighborMat(5,j)==1 && j~=5
        omegaij=stressMat(5,j);
        vx5=vx5-ka*kb*omegaij*(reP(1,5)-reP(1,j))-kb*omegaij*(reV(1,5)-reV(1,j));
        vy5=vy5-ka*kb*omegaij*(reP(2,5)-reP(2,j))-kb*omegaij*(reV(2,5)-reV(2,j));
    end
end
vx5=vx5+reV(1,5);
vy5=vy5+reV(2,5);


vx = vx5;
vy = vy5;

== matlab function GitAffineFormationDelayInput/Subsystem4/MATLAB Function12 ==
  data: deltaPfx output; p input; deltaPfy output
function [deltaPfx,deltaPfy]  = fcn_errorV4(p)

dim=2;
leaderNum=3;
stressMat=[-0.438878870659884,0.292585913773256,0.292585913773256,0,0,0,0,-0.0731464784433140,-0.0731464784433141;0.292585913773256,-0.615360326958201,0,0.420303051109364,-0.0673401385127307,0,-0.0301884994116881,0,0;0.292585913773256,0,-0.615360326958201,-0.0673401385127306,0.420303051109363,-0.0301884994116881,0,0,0;0,0.420303051109364,-0.0673401385127306,-0.703215455187769,-0.00271037000549659,0.352962912596633,0,0,0;0,-0.0673401385127307,0.420303051109363,-0.00271037000549659,-0.703215455187768,0,0.352962912596632,0,0;0,0,-0.0301884994116881,0.352962912596633,0,-0.607698639186239,-0.00766168777196264,0.292585913773257,0;0,-0.0301884994116881,0,0,0.352962912596632,-0.00766168777196264,-0.607698639186238,0,0.292585913773256;-0.0731464784433140,0,0,0,0,0.292585913773257,0,-0.402305631438228,0.182866196108285;-0.0731464784433141,0,0,0,0,0,0.292585913773256,0.182866196108285,-0.402305631438227];

stressMat_ff=stressMat(leaderNum+1:end,leaderNum+1:end);
stressMat_fl=stressMat(leaderNum+1:end,1:leaderNum);

p_all = p;
p_ell=p_all(1:dim*leaderNum);
p_f=p_all(dim*leaderNum+1:end);


delta=p_f+(kron(stressMat_ff,eye(dim)))\kron(stressMat_fl,eye(dim))*p_ell;
%deltaPf=delta(1,1)+delta(2,1);
deltaPfx=delta(9,1);
deltaPfy=delta(10,1);

== matlab function GitAffineFormationDelayInput/Subsystem5/MATLAB Function13 ==
  data: v input; vx output size=1; p input; vy output size=1; kaa input; kbb input
function [vx,vy] = fcn_followerV4(v,p,kaa,kbb)

reV=zeros(2,9);
reP=zeros(2,9);
reV=reshape(v,2,9);
reP=reshape(p,2,9);

ka=kaa;
kb=kbb;
vx9=0;
vy9=0;
nodenum=9;
leaderNum=3;
neighborMat=zeros(nodenum,nodenum);
neighborMat(1,2)=1;neighborMat(1,3)=1;neighborMat(1,8)=1;neighborMat(1,9)=1;
neighborMat(2,4)=1;neighborMat(2,7)=1;
neighborMat(3,5)=1;neighborMat(3,6)=1;neighborMat(3,4)=1;neighborMat(2,5)=1;
neighborMat(4,5)=1;neighborMat(4,6)=1;neighborMat(2,7)=1;neighborMat(4,7)=0;
neighborMat(5,7)=1;neighborMat(5,8)=0;neighborMat(5,6)=0;
neighborMat(6,7)=1;neighborMat(6,8)=1;
neighborMat(7,9)=1;
neighborMat(8,9)=1;
m=sum(sum(neighborMat)); % number of edges
neighborMat=neighborMat+neighborMat';
stressMat=[-0.438878870659884,0.292585913773256,0.292585913773256,0,0,0,0,-0.0731464784433140,-0.0731464784433141;0.292585913773256,-0.615360326958201,0,0.420303051109364,-0.0673401385127307,0,-0.0301884994116881,0,0;0.292585913773256,0,-0.615360326958201,-0.0673401385127306,0.420303051109363,-0.0301884994116881,0,0,0;0,0.420303051109364,-0.0673401385127306,-0.703215455187769,-0.00271037000549659,0.352962912596633,0,0,0;0,-0.0673401385127307,0.420303051109363,-0.00271037000549659,-0.703215455187768,0,0.352962912596632,0,0;0,0,-0.0301884994116881,0.352962912596633,0,-0.607698639186239,-0.00766168777196264,0.292585913773257,0;0,-0.0301884994116881,0,0,0.352962912596632,-0.00766168777196264,-0.607698639186238,0,0.292585913773256;-0.0731464784433140,0,0,0,0,0.292585913773257,0,-0.402305631438228,0.182866196108285;-0.0731464784433141,0,0,0,0,0,0.292585913773256,0.182866196108285,-0.402305631438227];

for j=1:nodenum 
    if neighborMat(9,j)==1 && j~=9
        omegaij=stressMat(9,j);
        vx9=vx9-ka*kb*omegaij*(reP(1,9)-reP(1,j))-kb*omegaij*(reV(1,9)-reV(1,j));
        vy9=vy9-ka*kb*omegaij*(reP(2,9)-reP(2,j))-kb*omegaij*(reV(2,9)-reV(2,j));
    end
end
vx9=vx9+reV(1,9);
vy9=vy9+reV(2,9);

vx = vx9;
vy = vy9;

== matlab function GitAffineFormationDelayInput/Subsystem5/MATLAB Function14 ==
  data: deltaPfx output; p input; deltaPfy output
function [deltaPfx,deltaPfy]  = fcn_errorV4(p)
leaderNum=3;
dim=2;
stressMat=[-0.438878870659884,0.292585913773256,0.292585913773256,0,0,0,0,-0.0731464784433140,-0.0731464784433141;0.292585913773256,-0.615360326958201,0,0.420303051109364,-0.0673401385127307,0,-0.0301884994116881,0,0;0.292585913773256,0,-0.615360326958201,-0.0673401385127306,0.420303051109363,-0.0301884994116881,0,0,0;0,0.420303051109364,-0.0673401385127306,-0.703215455187769,-0.00271037000549659,0.352962912596633,0,0,0;0,-0.0673401385127307,0.420303051109363,-0.00271037000549659,-0.703215455187768,0,0.352962912596632,0,0;0,0,-0.0301884994116881,0.352962912596633,0,-0.607698639186239,-0.00766168777196264,0.292585913773257,0;0,-0.0301884994116881,0,0,0.352962912596632,-0.00766168777196264,-0.607698639186238,0,0.292585913773256;-0.0731464784433140,0,0,0,0,0.292585913773257,0,-0.402305631438228,0.182866196108285;-0.0731464784433141,0,0,0,0,0,0.292585913773256,0.182866196108285,-0.402305631438227];
 
stressMat_ff=stressMat(leaderNum+1:end,leaderNum+1:end);
stressMat_fl=stressMat(leaderNum+1:end,1:leaderNum);

p_all = p;
p_ell=p_all(1:dim*leaderNum);
p_f=p_all(dim*leaderNum+1:end);


delta=p_f+(kron(stressMat_ff,eye(dim)))\kron(stressMat_fl,eye(dim))*p_ell;
%deltaPf=delta(1,1)+delta(2,1);
deltaPfx=delta(11,1);
deltaPfy=delta(12,1);

== matlab function GitAffineFormationDelayInput/Subsystem6/Subsystem15/MATLAB Function7 ==
  data: Vx input; vel output; Vy input; angle output; preangle input
function [vel,angle] = refer2carframe(Vx,Vy,preangle)
vel= sqrt(Vx^2+Vy^2);
  

if Vx > 0 && Vy > 0 
    angle = atan(Vy/Vx);
elseif Vx < 0 && Vy > 0 
    angle = pi+atan(Vy/Vx);
elseif Vx < 0 && Vy < 0 
    angle = pi+atan(Vy/Vx);
else
    angle = 2*pi+atan(Vy/Vx);
end

if Vx == 0 && Vy > 0
    angle = pi/2;
end
if Vx == 0 && Vy < 0
    angle = -pi/2;
end    
if Vx == 0 && Vy == 0
    angle = preangle;
end   
if Vy == 0 && Vx > 0
    angle = 0;
end
if Vy == 0 && Vx < 0
    angle = -pi;
end 

end

== matlab function GitAffineFormationDelayInput/Subsystem6/Subsystem15/MATLAB Function8 ==
  data: vel input; vx output; angle input; vy output
function [vx,vy] = unicycle(vel,angle)

vx=vel*cos(angle);
vy=vel*sin(angle);  

end

== matlab function GitAffineFormationDelayInput/Subsystem6/Subsystem15/MATLAB Function3 ==
  data: Vx input; vel output; Vy input; angle output; preangle input
function [vel,angle] = refer2carframe(Vx,Vy,preangle)
vel= sqrt(Vx^2+Vy^2);
  

if Vx > 0 && Vy > 0 
    angle = atan(Vy/Vx);
elseif Vx < 0 && Vy > 0 
    angle = pi+atan(Vy/Vx);
elseif Vx < 0 && Vy < 0 
    angle = pi+atan(Vy/Vx);
else
    angle = 2*pi+atan(Vy/Vx);
end

if Vx == 0 && Vy > 0
    angle = pi/2;
end
if Vx == 0 && Vy < 0
    angle = -pi/2;
end    
if Vx == 0 && Vy == 0
    angle = preangle;
end   
if Vy == 0 && Vx > 0
    angle = 0;
end
if Vy == 0 && Vx < 0
    angle = -pi;
end 

end

== matlab function GitAffineFormationDelayInput/Subsystem6/Subsystem15/MATLAB Function4 ==
  data: vel input; vx output; angle input; vy output
function [vx,vy] = unicycle(vel,angle)

vx=vel*cos(angle);
vy=vel*sin(angle);  

end

== matlab function GitAffineFormationDelayInput/Subsystem6/Subsystem15/MATLAB Function5 ==
  data: Vx input; vel output; Vy input; angle output; preangle input
function [vel,angle] = refer2carframe(Vx,Vy,preangle)
vel= sqrt(Vx^2+Vy^2);
  

if Vx > 0 && Vy > 0 
    angle = atan(Vy/Vx);
elseif Vx < 0 && Vy > 0 
    angle = pi+atan(Vy/Vx);
elseif Vx < 0 && Vy < 0 
    angle = pi+atan(Vy/Vx);
else
    angle = 2*pi+atan(Vy/Vx);
end

if Vx == 0 && Vy > 0
    angle = pi/2;
end
if Vx == 0 && Vy < 0
    angle = -pi/2;
end    
if Vx == 0 && Vy == 0
    angle = preangle;
end   
if Vy == 0 && Vx > 0
    angle = 0;
end
if Vy == 0 && Vx < 0
    angle = -pi;
end 

end

== matlab function GitAffineFormationDelayInput/Subsystem6/Subsystem15/MATLAB Function6 ==
  data: vel input; vx output; angle input; vy output
function [vx,vy] = unicycle(vel,angle)

vx=vel*cos(angle);
vy=vel*sin(angle);  

end

== matlab function GitAffineFormationDelayInput/Subsystem6/Subsystem15/MATLAB Function10 ==
  data: vel input; vx output; angle input; vy output
function [vx,vy] = unicycle(vel,angle)

vx=vel*cos(angle);
vy=vel*sin(angle);  

end

== matlab function GitAffineFormationDelayInput/Subsystem6/Subsystem15/MATLAB Function9 ==
  data: Vx input; vel output; Vy input; angle output; preangle input
function [vel,angle] = refer2carframe(Vx,Vy,preangle)
vel= sqrt(Vx^2+Vy^2);
  

if Vx > 0 && Vy > 0 
    angle = atan(Vy/Vx);
elseif Vx < 0 && Vy > 0 
    angle = pi+atan(Vy/Vx);
elseif Vx < 0 && Vy < 0 
    angle = pi+atan(Vy/Vx);
else
    angle = 2*pi+atan(Vy/Vx);
end

if Vx == 0 && Vy > 0
    angle = pi/2;
end
if Vx == 0 && Vy < 0
    angle = -pi/2;
end    
if Vx == 0 && Vy == 0
    angle = preangle;
end   
if Vy == 0 && Vx > 0
    angle = 0;
end
if Vy == 0 && Vx < 0
    angle = -pi;
end 

end

== matlab function GitAffineFormationDelayInput/Subsystem1/MATLAB Function6 ==
  data: deltaPfx output; p input; deltaPfy output
function [deltaPfx,deltaPfy]  = fcn_errorV4(p)

leaderNum=3;
dim=2;
stressMat=[-0.438878870659884,0.292585913773256,0.292585913773256,0,0,0,0,-0.0731464784433140,-0.0731464784433141;0.292585913773256,-0.615360326958201,0,0.420303051109364,-0.0673401385127307,0,-0.0301884994116881,0,0;0.292585913773256,0,-0.615360326958201,-0.0673401385127306,0.420303051109363,-0.0301884994116881,0,0,0;0,0.420303051109364,-0.0673401385127306,-0.703215455187769,-0.00271037000549659,0.352962912596633,0,0,0;0,-0.0673401385127307,0.420303051109363,-0.00271037000549659,-0.703215455187768,0,0.352962912596632,0,0;0,0,-0.0301884994116881,0.352962912596633,0,-0.607698639186239,-0.00766168777196264,0.292585913773257,0;0,-0.0301884994116881,0,0,0.352962912596632,-0.00766168777196264,-0.607698639186238,0,0.292585913773256;-0.0731464784433140,0,0,0,0,0.292585913773257,0,-0.402305631438228,0.182866196108285;-0.0731464784433141,0,0,0,0,0,0.292585913773256,0.182866196108285,-0.402305631438227];


%stressMat=fcn_StressMatrix(2,nodenum,m,P,neighborMat); 
stressMat_ff=stressMat(leaderNum+1:end,leaderNum+1:end);
stressMat_fl=stressMat(leaderNum+1:end,1:leaderNum);

p_all = p;
p_ell=p_all(1:dim*leaderNum);
p_f=p_all(dim*leaderNum+1:end);


delta=p_f+(kron(stressMat_ff,eye(dim)))\kron(stressMat_fl,eye(dim))*p_ell;
%deltaPf=delta(1,1)+delta(2,1);
deltaPfx=delta(3,1);
deltaPfy=delta(4,1);

== matlab function GitAffineFormationDelayInput/Subsystem6/Subsystem15/MATLAB Function11 ==
  data: Vx input; vel output; Vy input; angle output; preangle input
function [vel,angle] = refer2carframe(Vx,Vy,preangle)
vel= sqrt(Vx^2+Vy^2);
  

if Vx > 0 && Vy > 0 
    angle = atan(Vy/Vx);
elseif Vx < 0 && Vy > 0 
    angle = pi+atan(Vy/Vx);
elseif Vx < 0 && Vy < 0 
    angle = pi+atan(Vy/Vx);
else
    angle = 2*pi+atan(Vy/Vx);
end

if Vx == 0 && Vy > 0
    angle = pi/2;
end
if Vx == 0 && Vy < 0
    angle = -pi/2;
end    
if Vx == 0 && Vy == 0
    angle = preangle;
end   
if Vy == 0 && Vx > 0
    angle = 0;
end
if Vy == 0 && Vx < 0
    angle = -pi;
end 

end

== matlab function GitAffineFormationDelayInput/Subsystem6/Subsystem15/MATLAB Function12 ==
  data: vel input; vx output; angle input; vy output
function [vx,vy] = unicycle(vel,angle)

vx=vel*cos(angle);
vy=vel*sin(angle);  

end

== matlab function GitAffineFormationDelayInput/Subsystem6/Subsystem15/MATLAB Function13 ==
  data: Vx input; vel output; Vy input; angle output; preangle input
function [vel,angle] = refer2carframe(Vx,Vy,preangle)
vel= sqrt(Vx^2+Vy^2);
  

if Vx > 0 && Vy > 0 
    angle = atan(Vy/Vx);
elseif Vx < 0 && Vy > 0 
    angle = pi+atan(Vy/Vx);
elseif Vx < 0 && Vy < 0 
    angle = pi+atan(Vy/Vx);
else
    angle = 2*pi+atan(Vy/Vx);
end

if Vx == 0 && Vy > 0
    angle = pi/2;
end
if Vx == 0 && Vy < 0
    angle = -pi/2;
end    
if Vx == 0 && Vy == 0
    angle = preangle;
end   
if Vy == 0 && Vx > 0
    angle = 0;
end
if Vy == 0 && Vx < 0
    angle = -pi;
end 

end

== matlab function GitAffineFormationDelayInput/Subsystem6/Subsystem15/MATLAB Function14 ==
  data: vel input; vx output; angle input; vy output
function [vx,vy] = unicycle(vel,angle)

vx=vel*cos(angle);
vy=vel*sin(angle);  

end

== matlab function GitAffineFormationDelayInput/Subsystem6/Subsystem15/MATLAB Function15 ==
  data: Vx input; vel output; Vy input; angle output; preangle input
function [vel,angle] = refer2carframe(Vx,Vy,preangle)
vel= sqrt(Vx^2+Vy^2);
  

if Vx > 0 && Vy > 0 
    angle = atan(Vy/Vx);
elseif Vx < 0 && Vy > 0 
    angle = pi+atan(Vy/Vx);
elseif Vx < 0 && Vy < 0 
    angle = pi+atan(Vy/Vx);
else
    angle = 2*pi+atan(Vy/Vx);
end

if Vx == 0 && Vy > 0
    angle = pi/2;
end
if Vx == 0 && Vy < 0
    angle = -pi/2;
end    
if Vx == 0 && Vy == 0
    angle = preangle;
end   
if Vy == 0 && Vx > 0
    angle = 0;
end
if Vy == 0 && Vx < 0
    angle = -pi;
end 

end

== matlab function GitAffineFormationDelayInput/Subsystem6/Subsystem15/MATLAB Function16 ==
  data: vel input; vx output; angle input; vy output
function [vx,vy] = unicycle(vel,angle)

vx=vel*cos(angle);
vy=vel*sin(angle);  

end

== matlab function GitAffineFormationDelayInput/Subsystem6/Subsystem15/MATLAB Function17 ==
  data: Vx input; vel output; Vy input; angle output; preangle input
function [vel,angle] = refer2carframe(Vx,Vy,preangle)
vel= sqrt(Vx^2+Vy^2);
  

if Vx > 0 && Vy > 0 
    angle = atan(Vy/Vx);
elseif Vx < 0 && Vy > 0 
    angle = pi+atan(Vy/Vx);
elseif Vx < 0 && Vy < 0 
    angle = pi+atan(Vy/Vx);
else
    angle = 2*pi+atan(Vy/Vx);
end

if Vx == 0 && Vy > 0
    angle = pi/2;
end
if Vx == 0 && Vy < 0
    angle = -pi/2;
end    
if Vx == 0 && Vy == 0
    angle = preangle;
end   
if Vy == 0 && Vx > 0
    angle = 0;
end
if Vy == 0 && Vx < 0
    angle = -pi;
end 

end

== matlab function GitAffineFormationDelayInput/Subsystem6/Subsystem15/MATLAB Function18 ==
  data: vel input; vx output; angle input; vy output
function [vx,vy] = unicycle(vel,angle)

vx=vel*cos(angle);
vy=vel*sin(angle);  

end

== matlab function GitAffineFormationDelayInput/Subsystem6/Subsystem15/MATLAB Function19 ==
  data: Vx input; vel output; Vy input; angle output; preangle input
function [vel,angle] = refer2carframe(Vx,Vy,preangle)
vel= sqrt(Vx^2+Vy^2);
  

if Vx > 0 && Vy > 0 
    angle = atan(Vy/Vx);
elseif Vx < 0 && Vy > 0 
    angle = pi+atan(Vy/Vx);
elseif Vx < 0 && Vy < 0 
    angle = pi+atan(Vy/Vx);
else
    angle = 2*pi+atan(Vy/Vx);
end

if Vx == 0 && Vy > 0
    angle = pi/2;
end
if Vx == 0 && Vy < 0
    angle = -pi/2;
end    
if Vx == 0 && Vy == 0
    angle = preangle;
end   
if Vy == 0 && Vx > 0
    angle = 0;
end
if Vy == 0 && Vx < 0
    angle = -pi;
end 

end

== matlab function GitAffineFormationDelayInput/Subsystem2/MATLAB Function7 ==
  data: v input; vx output size=1; p input; vy output size=1; kaa input; kbb input
function [vx,vy] = fcn_followerV4(v,p,kaa,kbb)

reV=zeros(2,9);
reP=zeros(2,9);
reV=reshape(v,2,9);
reP=reshape(p,2,9);

ka=kaa;
kb=kbb;
vx6=0;
vy6=0;
nodenum=9;
leaderNum=3;
neighborMat=zeros(nodenum,nodenum);
neighborMat(1,2)=1;neighborMat(1,3)=1;neighborMat(1,8)=1;neighborMat(1,9)=1;
neighborMat(2,4)=1;neighborMat(2,7)=1;
neighborMat(3,5)=1;neighborMat(3,6)=1;neighborMat(3,4)=1;neighborMat(2,5)=1;
neighborMat(4,5)=1;neighborMat(4,6)=1;neighborMat(2,7)=1;neighborMat(4,7)=0;
neighborMat(5,7)=1;neighborMat(5,8)=0;neighborMat(5,6)=0;
neighborMat(6,7)=1;neighborMat(6,8)=1;
neighborMat(7,9)=1;
neighborMat(8,9)=1;
m=sum(sum(neighborMat)); % number of edges
neighborMat=neighborMat+neighborMat';
stressMat=[-0.438878870659884,0.292585913773256,0.292585913773256,0,0,0,0,-0.0731464784433140,-0.0731464784433141;0.292585913773256,-0.615360326958201,0,0.420303051109364,-0.0673401385127307,0,-0.0301884994116881,0,0;0.292585913773256,0,-0.615360326958201,-0.0673401385127306,0.420303051109363,-0.0301884994116881,0,0,0;0,0.420303051109364,-0.0673401385127306,-0.703215455187769,-0.00271037000549659,0.352962912596633,0,0,0;0,-0.0673401385127307,0.420303051109363,-0.00271037000549659,-0.703215455187768,0,0.352962912596632,0,0;0,0,-0.0301884994116881,0.352962912596633,0,-0.607698639186239,-0.00766168777196264,0.292585913773257,0;0,-0.0301884994116881,0,0,0.352962912596632,-0.00766168777196264,-0.607698639186238,0,0.292585913773256;-0.0731464784433140,0,0,0,0,0.292585913773257,0,-0.402305631438228,0.182866196108285;-0.0731464784433141,0,0,0,0,0,0.292585913773256,0.182866196108285,-0.402305631438227];

for j=1:nodenum 
    if neighborMat(6,j)==1 && j~=6
        omegaij=stressMat(6,j);
        vx6=vx6-ka*kb*omegaij*(reP(1,6)-reP(1,j))-kb*omegaij*(reV(1,6)-reV(1,j));
        vy6=vy6-ka*kb*omegaij*(reP(2,6)-reP(2,j))-kb*omegaij*(reV(2,6)-reV(2,j));
    end
end
vx6=vx6+reV(1,6);
vy6=vy6+reV(2,6);
vx = vx6;
vy = vy6;

== matlab function GitAffineFormationDelayInput/Subsystem6/Subsystem15/MATLAB Function20 ==
  data: vel input; vx output; angle input; vy output
function [vx,vy] = unicycle(vel,angle)

vx=vel*cos(angle);
vy=vel*sin(angle);  

end

== matlab function GitAffineFormationDelayInput/Subsystem2/MATLAB Function8 ==
  data: deltaPfx output; p input; deltaPfy output
function [deltaPfx,deltaPfy]  = fcn_errorV4(p)
leaderNum=3;
dim=2;
stressMat=[-0.438878870659884,0.292585913773256,0.292585913773256,0,0,0,0,-0.0731464784433140,-0.0731464784433141;0.292585913773256,-0.615360326958201,0,0.420303051109364,-0.0673401385127307,0,-0.0301884994116881,0,0;0.292585913773256,0,-0.615360326958201,-0.0673401385127306,0.420303051109363,-0.0301884994116881,0,0,0;0,0.420303051109364,-0.0673401385127306,-0.703215455187769,-0.00271037000549659,0.352962912596633,0,0,0;0,-0.0673401385127307,0.420303051109363,-0.00271037000549659,-0.703215455187768,0,0.352962912596632,0,0;0,0,-0.0301884994116881,0.352962912596633,0,-0.607698639186239,-0.00766168777196264,0.292585913773257,0;0,-0.0301884994116881,0,0,0.352962912596632,-0.00766168777196264,-0.607698639186238,0,0.292585913773256;-0.0731464784433140,0,0,0,0,0.292585913773257,0,-0.402305631438228,0.182866196108285;-0.0731464784433141,0,0,0,0,0,0.292585913773256,0.182866196108285,-0.402305631438227]; 
stressMat_ff=stressMat(leaderNum+1:end,leaderNum+1:end);
stressMat_fl=stressMat(leaderNum+1:end,1:leaderNum);

p_all = p;
p_ell=p_all(1:dim*leaderNum);
p_f=p_all(dim*leaderNum+1:end);


delta=p_f+(kron(stressMat_ff,eye(dim)))\kron(stressMat_fl,eye(dim))*p_ell;
%deltaPf=delta(1,1)+delta(2,1);
deltaPfx=delta(5,1);
deltaPfy=delta(6,1);

== matlab function GitAffineFormationDelayInput/Subsystem3/MATLAB Function10 ==
  data: deltaPfx output; p input; deltaPfy output
function [deltaPfx,deltaPfy]  = fcn_errorV4(p)

leaderNum=3;
dim=2;
stressMat=[-0.438878870659884,0.292585913773256,0.292585913773256,0,0,0,0,-0.0731464784433140,-0.0731464784433141;0.292585913773256,-0.615360326958201,0,0.420303051109364,-0.0673401385127307,0,-0.0301884994116881,0,0;0.292585913773256,0,-0.615360326958201,-0.0673401385127306,0.420303051109363,-0.0301884994116881,0,0,0;0,0.420303051109364,-0.0673401385127306,-0.703215455187769,-0.00271037000549659,0.352962912596633,0,0,0;0,-0.0673401385127307,0.420303051109363,-0.00271037000549659,-0.703215455187768,0,0.352962912596632,0,0;0,0,-0.0301884994116881,0.352962912596633,0,-0.607698639186239,-0.00766168777196264,0.292585913773257,0;0,-0.0301884994116881,0,0,0.352962912596632,-0.00766168777196264,-0.607698639186238,0,0.292585913773256;-0.0731464784433140,0,0,0,0,0.292585913773257,0,-0.402305631438228,0.182866196108285;-0.0731464784433141,0,0,0,0,0,0.292585913773256,0.182866196108285,-0.402305631438227];

stressMat_ff=stressMat(leaderNum+1:end,leaderNum+1:end);
stressMat_fl=stressMat(leaderNum+1:end,1:leaderNum);

p_all = p;
p_ell=p_all(1:dim*leaderNum);
p_f=p_all(dim*leaderNum+1:end);


delta=p_f+(kron(stressMat_ff,eye(dim)))\kron(stressMat_fl,eye(dim))*p_ell;
%deltaPf=delta(1,1)+delta(2,1);
deltaPfx=delta(7,1);
deltaPfy=delta(8,1);
